simulink model "accBasedController_2015a"  (Simulink 8.5)
settings: Solver=ode45  SolverMode=SingleTasking  StartTime=0.0  StopTime=6  FixedStep=0.001  RelTol=1e-3
values from neighbouring files (symbols this model uses):
  A = [0 0 0 1 0 0;      0 0 0 0 1 0;      0 0 0 0 0 1;      -Ka/Jh Ka/Jh 0 0 0 0;     Ka/Je -(Ks + Ka)/Je Ks/Je 0 0 0;      0 Ks/Ja -Ks/Ja 0 0 -Beq/Ja]    [SimulationParam.m]    (also in SimulationParameters.m; abc_ws.mat = [0 0 0 1567.93947765 0 0 0 0 -1685.45584092 221.276595745 0 ; kalmanSS.m = [0 0 0 1 0 0;      0 0 0 0 1 0;      0 0 0 0 0 1;      -Ka/J; kalmanSSHumInput.m = [zeros(1,state_dim);      0 0 0 1 0;      0 0 0 0 1;      Ka)
  B = [zeros(3,control_dim); 1/Jh 0 0; 0 -1/Je 0; 0 0 N*KI/Ja]    [SimulationParam.m]    (also in SimulationParameters.m; abc_ws.mat = [1 0 0 0 0 0 0 0 -1.12996503145 0 0 0 ... (15 elements, 5x3); kalmanSS.m; kalmanSSHumInput.m = [1 0 0; zeros(2,control_dim); 0 -1/Je 0; 0 0 N*KI/Ja])
  Beq = 60    [SimulationParam.m]    (also in SimulationParameters.m; abc_ws.mat; kalmanSS.m; kalmanSSHumInput.m)
  C = [zeros(sensor_dim,state_dim)]    [SimulationParam.m]    (also in SimulationParameters.m; abc_ws.mat = [-1387.6 0 0 0 0 0 1387.6 0 1 0 0 0 ... (30 elements, 6x5)]; kalmanSS.m; kalmanSSHumInput.m)
  CURRENT_MAX = pi    (= 3.14159265359)    [SimulationParam.m]    (also in SimulationParameters.m; abc_ws.mat = 3.14)
  D = zeros(sensor_dim, control_dim)    [SimulationParam.m]    (also in SimulationParameters.m; abc_ws.mat = [0 1 0 0 0 0 0 0 0 0 0 0 ... (18 elements, 6x3)]; kalmanSS.m; kalmanSSHumInput.m = zeros(sensor_dim, control_dim); D(2,1) = 1)
  f = logspace(-2,2,1e4)    [kalmanSSHumInput.m]
  Ja = 0.47    [SimulationParam.m]    (also in SimulationParameters.m; abc_ws.mat; kalmanSS.m; kalmanSSHumInput.m)
  Je = W*Le^2    (= 0.88498313856)    [SimulationParam.m]    (also in SimulationParameters.m; abc_ws.mat; kalmanSS.m; kalmanSSHumInput.m)
  KI = 0.0603    [SimulationParam.m]    (also in SimulationParameters.m; abc_ws.mat; kalmanSS.m; kalmanSSHumInput.m)
  Le = 0.432    [SimulationParam.m]    (also in SimulationParameters.m; abc_ws.mat; kalmanSS.m; kalmanSSHumInput.m)
  N = 150    [SimulationParam.m]    (also in SimulationParameters.m; abc_ws.mat; kalmanSS.m; kalmanSSHumInput.m)
  Threaded_Ts = 0.001    [SimulationParam.m]    (also in SimulationParameters.m; abc_ws.mat)
  We = W*g    (= 46.5037717323)    [SimulationParam.m]    (also in SimulationParameters.m; abc_ws.mat; kalmanSS.m; kalmanSSHumInput.m)
libraries: simulink_extras x4, simulink x3, instrumentlib x2, eeGeneralControl x1
Description:
  | Collocated Admittance Control study for the acceleration-based SEA Transparency Control
settings Model: Creator=Leonardo Felipe  LastModifiedBy=leona  CovMetricSettings=dwe  CovHtmlReporting=off  covSaveCumulativeToWorkspaceVar=off  CovSaveSingleToWorkspaceVar=off  CovExternalEMLEnable=on
settings DataIOCC: MaxDataPoints=23000  SignalLoggingSaveFormat=Dataset  InspectSignalLogs=on
settings OptimizationCC: ExpressionDepthLimit=128
settings DebuggingCC: UnderspecifiedInitializationDetection=Simplified  MergeDetectMultiDrivingBlocksExec=error  FcnCallInpInsideContextMsg=EnableAllAsError  StateNameClashWarn=none  SFUnexpectedBacktrackingDiag=error  SFNoUnconditionalDefaultTransitionDiag=error
settings HardwareCC: ProdBitPerPointer=64  ProdLargestAtomicFloat=Float  ProdIntDivRoundTo=Zero  ProdEndianess=LittleEndian  ProdHWDeviceType=Specified
settings ModelReferenceCC: PropagateSignalLabelsOutOfModel=on
settings SFSimCC: SimUseLocalCustomCode=on
settings RTWCC: RTWUseLocalCustomCode=on
settings GRTTargetCC: TargetLangStandard=C99 (ISO)  CombineOutputUpdateFcns=on  GRTInterface=off

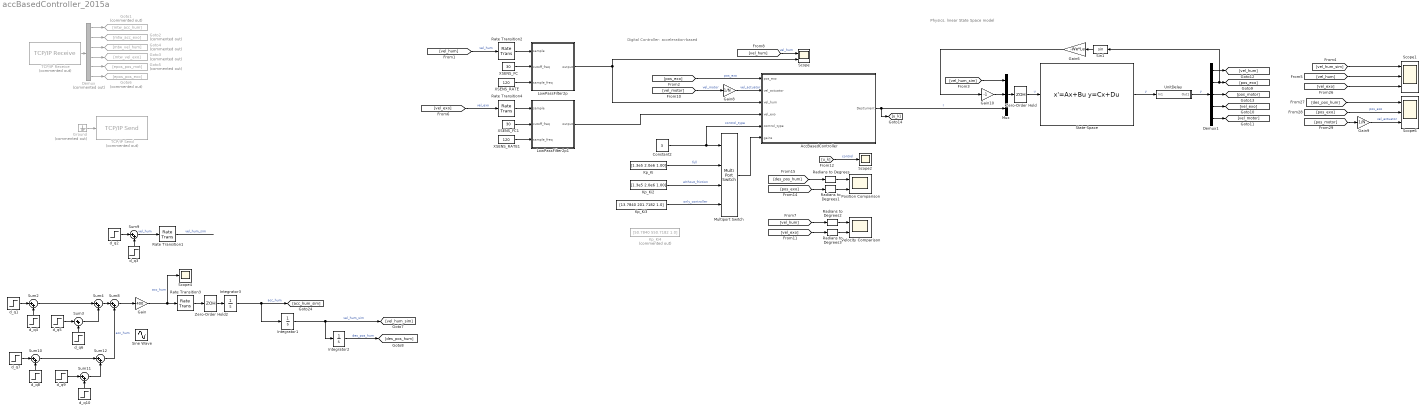
== system accBasedController_2015a ==
  note: Digital Controller: acceleration-based
  note: Physics, linear State Space model
  AccBasedController : Subsystem
  Constant2 : Constant  Value=3
  Demux : Demux  Commented=on  Outputs=6
  Demux1 : Demux  Outputs=5
  Gain : Gain  Gain=400
  Gain10 : Gain  Gain=-1
  Gain6 : Gain  Gain=-We*Le
  Gain8 : Gain  Gain=1/N
  Gain9 : Gain  Gain=1/N
  Goto1 : Goto  Commented=on  GotoTag=mtw_acc_hum
  Goto2 : Goto  Commented=on  GotoTag=mtw_acc_exo
  Goto3 : Goto  Commented=on  GotoTag=mtw_vel_exo
  Goto4 : Goto  Commented=on  GotoTag=mtw_vel_hum
  Goto5 : Goto  Commented=on  GotoTag=epos_pos_mot
  Goto6 : Goto  Commented=on  GotoTag=epos_pos_exo
  Ground : Ground  Commented=on
  Integrator1 : Integrator
  Integrator2 : Integrator
  Integrator3 : Integrator
  Kp_Ki : Constant  Value=[1.3e5 2.0e6 1.00]
  Kp_Ki2 : Constant  Value=[1.3e5 2.0e6 1.00]
  Kp_Ki3 : Constant  Value=[13.7840 201.7182 1.0]
  Kp_Ki4 : Constant  Commented=on  Value=[50.7840 550.7182 1.0]
  LowPassFilter2p : Subsystem
  LowPassFilter2p1 : Subsystem
  Multiport Switch : MultiPortSwitch
  Mux : Mux  Inputs=3
  Position Comparison : Scope  NumInputPorts=2
      settings: TimeRange=auto  MaxDataPoints=5000  SaveToWorkspace=off  YMin=-3.29771~-5  YMax=29.67935~5  SampleTime=-1
  Radians to Degrees{,1..3} (4 alike) : simulink_extras/Transformations/Radians to Degrees
  Rate Transition1 : RateTransition  OutPortSampleTime=Threaded_Ts
  Rate Transition2 : RateTransition  OutPortSampleTime=0.008
  Rate Transition3 : RateTransition  OutPortSampleTime=Threaded_Ts
  Rate Transition4 : RateTransition  OutPortSampleTime=0.008
  Scope : Scope  NumInputPorts=2
      settings: TimeRange=auto  MaxDataPoints=5000  SaveToWorkspace=off  SaveName=ScopeData2  YMin=-0.03282~-5  YMax=0.26283~5  SampleTime=-1
  Scope1 : Scope  NumInputPorts=3
      settings: TimeRange=auto  MaxDataPoints=5000  SaveToWorkspace=off  YMin=-0.01455~-5~-5  YMax=0.24273~5~5  SampleTime=-1
  Scope2 : Scope
      settings: TimeRange=auto  MaxDataPoints=5000  SaveToWorkspace=off  YMin=-3.925  YMax=3.925  SampleTime=-1
  Scope4 : Scope
      settings: TimeRange=auto  MaxDataPoints=5000  SaveToWorkspace=off  SaveName=ScopeData4  YMin=-50.00000  YMax=50.00000  SampleTime=-1
  Scope6 : Scope  NumInputPorts=3
      settings: TimeRange=auto  ShowLegends=on  MaxDataPoints=5000  SaveToWorkspace=off  YMin=-0.05756~-5~-5  YMax=0.518~5~5  SampleTime=-1
  Sin1 : Trigonometry
  Sine Wave : Sin  SampleTime=0
  State-Space : StateSpace  A=A  B=B  C=C  D=D  X0=0  ContinuousStateAttributes={'x_h','x_e','x_a','dx_e','dx_a'}
  Sum{2..4,8..12} (8 alike) : Sum  Inputs=|++
  TCP/IP Receive : instrumentlib/TCP//IP Receive  Commented=on  Host=127.0.0.1  Port=23000  DataSize="[1  6]"  EnableBlockingMode=on  Timeout=0.3  SampleTime=Threaded_Ts  DataType=single  ByteOrder=BigEndian  ASCIIFormatting=%f,  Terminator=LF
  TCP/IP Send : instrumentlib/TCP//IP Send  Commented=on  Host=127.0.0.1  Port=23001  EnableBlockingMode=on  Timeout=0.3  ByteOrder=BigEndian  TransferDelay=off
  UnitDelay : Subsystem  TreatAsAtomicUnit=on  SystemSampleTime=Threaded_Ts
  Velocity Comparison : Scope  NumInputPorts=2
      settings: TimeRange=auto  MaxDataPoints=5000  SaveToWorkspace=off  SaveName=ScopeData2  YMin=-7.82186~-5  YMax=13.60083~5  SampleTime=-1
  XSENS_FC : Constant  Value=30
  XSENS_FC1 : Constant  Value=30
  XSENS_RATE : Constant  Value=120
  XSENS_RATE1 : Constant  Value=120
  Zero-Order Hold : ZeroOrderHold  SampleTime=Threaded_Ts
  Zero-Order Hold2 : ZeroOrderHold  SampleTime=Threaded_Ts
  d_q1 : Step  Time=0.76  SampleTime=0.008
  d_q10 : Step  Time=2.808  After=-1  SampleTime=0.008
  d_q2 : Step  SampleTime=0.008
  d_q3 : Step  Time=1.4  After=-1  SampleTime=0.008
  d_q4 : Step  Time=0.784  After=-1  SampleTime=0.008
  d_q5 : Step  Time=0.784  After=-1  SampleTime=0.008
  d_q6 : Step  Time=0.808  SampleTime=0.008
  d_q7 : Step  Time=2.76  After=-1  SampleTime=0.008
  d_q8 : Step  Time=2.784  SampleTime=0.008
  d_q9 : Step  Time=2.784  SampleTime=0.008
  wires:
  d_q3/1 -> Sum9/2
  d_q2/1 -> Sum9/1
  Sum9/1 -> Rate Transition1/1  "vel_hum"
  TCP/IP Receive/1 -> Demux/1
  Demux/1 -> Goto1/1
  Demux/2 -> Goto2/1
  Demux/3 -> Goto4/1
  Demux/4 -> Goto3/1
  Demux/5 -> Goto5/1
  Demux/6 -> Goto6/1
  Ground/1 -> TCP/IP Send/1
  Integrator1/1 -> Integrator2/1, [vel_hum_sim]  "vel_hum_sim"
  Integrator2/1 -> [des_pos_hum]  "des_pos_hum"
  Zero-Order Hold/1 -> State-Space/1  "u"
  State-Space/1 -> UnitDelay/1(In1)  "y"
  [vel_hum_sim] -> Mux/1
  Mux/1 -> Zero-Order Hold/1
  Demux1/5 -> [vel_motor]
  Demux1/1 -> [vel_hum]
  UnitDelay/1(Out1) -> Demux1/1  "y"
  [vel_hum_sim] -> Scope1/1
  [vel_hum] -> Scope1/2
  [vel_hum] -> Radians to Degrees2/1
  [vel_exo] -> Radians to Degrees3/1
  [des_pos_hum] -> Radians to Degrees/1
  [pos_exo] -> Radians to Degrees1/1
  d_q1/1 -> Sum2/1
  d_q4/1 -> Sum2/2
  d_q6/1 -> Sum3/2
  d_q5/1 -> Sum3/1
  Sum2/1 -> Sum4/1
  Sum3/1 -> Sum4/2
  Sum8/1 -> Gain/1
  Rate Transition1/1 -> ?  "vel_hum_sim"
  Zero-Order Hold2/1 -> Integrator3/1
  Integrator3/1 -> Integrator1/1, [acc_hum_sim]  "acc_hum"
  Rate Transition3/1 -> Zero-Order Hold2/1
  Sum11/1 -> Sum12/2
  Sum10/1 -> Sum12/1
  d_q9/1 -> Sum11/1
  d_q10/1 -> Sum11/2
  d_q8/1 -> Sum10/2
  d_q7/1 -> Sum10/1
  Sum4/1 -> Sum8/1
  Sum12/1 -> Sum8/2  "acc_hum"
  [vel_exo] -> Scope1/3
  [des_pos_hum] -> Scope6/1
  [pos_exo] -> Scope6/2  "pos_exo"
  Gain/1 -> Rate Transition3/1, Scope4/1  "acc_hum"
  Kp_Ki/1 -> Multiport Switch/2  "full"
  Kp_Ki2/1 -> Multiport Switch/3  "without_friction"
  Kp_Ki3/1 -> Multiport Switch/4  "only_controller"
  Constant2/1 -> AccBasedController/5(control_type), Multiport Switch/1  "control_type"
  [pos_exo] -> AccBasedController/1(pos_exo)  "pos_exo"
  [vel_motor] -> Gain8/1  "vel_motor"
  Multiport Switch/1 -> AccBasedController/6(gains)
  Sin1/1 -> Gain6/1
  Demux1/2 -> Sin1/1, [pos_exo]
  AccBasedController/1(DesCurrent) -> Mux/3, [u_k]  "I"
  Gain6/1 -> Gain10/1
  Demux1/3 -> [pos_motor]
  Demux1/4 -> [vel_exo]
  Gain8/1 -> AccBasedController/2(vel_actuator)  "vel_actuator"
  [pos_motor] -> Gain9/1
  Gain9/1 -> Scope6/3  "vel_actuator"
  Radians to Degrees/1 -> Position Comparison/1
  Radians to Degrees1/1 -> Position Comparison/2
  Radians to Degrees2/1 -> Velocity Comparison/1
  Radians to Degrees3/1 -> Velocity Comparison/2
  [u_k] -> Scope2/1  "control"
  Gain10/1 -> Mux/2
  Rate Transition2/1 -> LowPassFilter2p/1(sample)
  XSENS_RATE/1 -> LowPassFilter2p/3(sample_freq)
  XSENS_FC/1 -> LowPassFilter2p/2(cutoff_freq)
  [vel_hum] -> Scope/1  "vel_hum"
  [vel_hum] -> Rate Transition2/1  "vel_hum"
  LowPassFilter2p/1(output) -> AccBasedController/3(vel_hum), Scope/2
  XSENS_FC1/1 -> LowPassFilter2p1/2(cutoff_freq)
  XSENS_RATE1/1 -> LowPassFilter2p1/3(sample_freq)
  Rate Transition4/1 -> LowPassFilter2p1/1(sample)
  [vel_exo] -> Rate Transition4/1  "vel_exo"
  LowPassFilter2p1/1(output) -> AccBasedController/4(vel_exo)

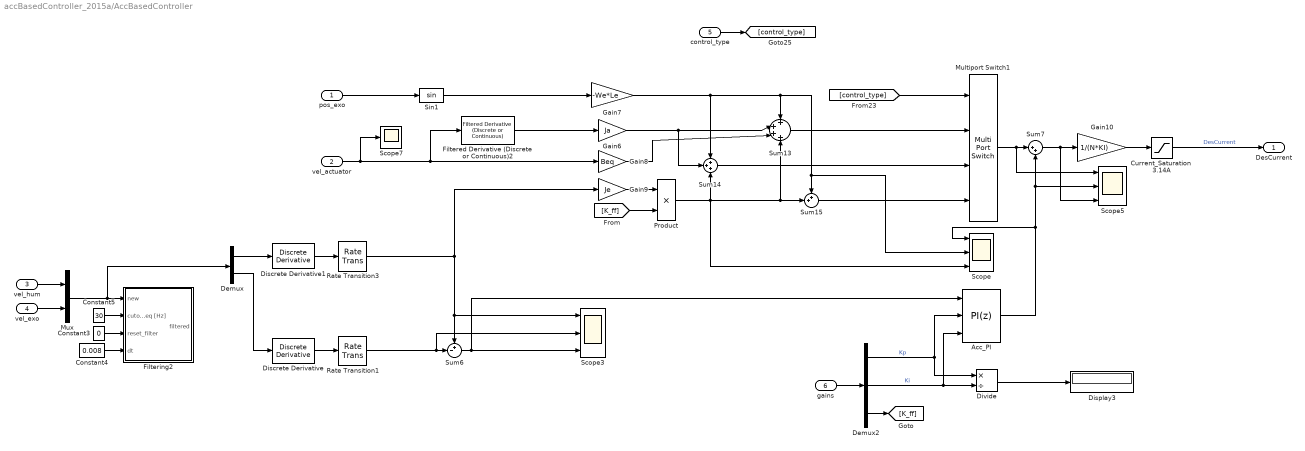
== system accBasedController_2015a/AccBasedController ==
  pos_exo : Inport
  vel_actuator : Inport  Port=2
  vel_hum : Inport  Port=3
  vel_exo : Inport  Port=4
  control_type : Inport  Port=5
  gains : Inport  Port=6
  Acc_PI : simulink/Continuous/PID Controller  Controller=PI  Form=Parallel  TimeDomain=Discrete-time  SampleTime=Threaded_Ts  IntegratorMethod=Forward Euler  FilterMethod=Forward Euler  ControllerParametersSource=external  P=13.7840  I=101.7182  D=0  UseFilter=on  N=100  InitialConditionSource=internal  InitialConditionForIntegrator=0  InitialConditionForFilter=0  DifferentiatorICPrevScaledInput=0  ExternalReset=none  TrackingMode=off  Kt=1  LimitOutput=off  UpperSaturationLimit=inf  LowerSaturationLimit=-inf  LinearizeAsGain=on  AntiWindupMode=none  Kb=1  POutMin=[]  POutMax=[]  IOutMin=[]  IOutMax=[]  DOutMin=[]  DOutMax=[]  NOutMin=[]  NOutMax=[]  SumOutMin=[]  SumOutMax=[]  SaturationOutMin=[]  SaturationOutMax=[]  PParamMin=[]  PParamMax=[]  IParamMin=[]  IParamMax=[]  DParamMin=[]  DParamMax=[]  NParamMin=[]  NParamMax=[]  KbParamMin=[]  KbParamMax=[]  KtParamMin=[]  KtParamMax=[]  KbOutMin=[]  KbOutMax=[]  KtOutMin=[]  KtOutMax=[]  IntegratorOutMin=[]  IntegratorOutMax=[]  FilterOutMin=[]  FilterOutMax=[]  SumI1OutMin=[]  SumI1OutMax=[]  SumI2OutMin=[]  SumI2OutMax=[]  SumI3OutMin=[]  SumI3OutMax=[]  SumDOutMin=[]  SumDOutMax=[]  DifferentiatorOutMin=[]  DifferentiatorOutMax=[]  IntegratorContinuousStateAttributes=''  IntegratorStateMustResolveToSignalObject=off  IntegratorRTWStateStorageClass=Auto  FilterContinuousStateAttributes=''  FilterStateMustResolveToSignalObject=off  FilterRTWStateStorageClass=Auto
  Constant3 : Constant  Value=0
  Constant4 : Constant  Value=0.008
  Constant5 : Constant  Value=30
  Current_Saturation  3.14A : Saturate  UpperLimit=CURRENT_MAX  LowerLimit=-CURRENT_MAX
  Demux : Demux  Outputs=2
  Demux2 : Demux  Outputs=3
  Discrete Derivative : simulink/Discrete/Discrete Derivative  gainval=1.0  ICPrevScaledInput=0.0  OutMin=[]  OutMax=[]  OutDataType=fixdt(1, 16)  OutScaling=2^-10  DoSatur=off
  Discrete Derivative1 : simulink/Discrete/Discrete Derivative  gainval=1.0  ICPrevScaledInput=0.0  OutMin=[]  OutMax=[]  OutDataType=fixdt(1, 16)  OutScaling=2^-10  DoSatur=off
  Display3 : Display
  Divide : Product  Inputs=*/
  Filtered Derivative (Discrete or Continuous)2 : eeGeneralControl/Filtered Derivative (Discrete or Continuous)  K=1  T=0.01  B=10000  A=-10000  minRatio=10  init_option=Inherited from block input  x0=0  Ts=Threaded_Ts
  Filtering2 : Subsystem
  Gain10 : Gain  Gain=1/(N*KI)
  Gain6 : Gain  Gain=Ja
  Gain7 : Gain  Gain=-We*Le
  Gain8 : Gain  Gain=Beq
  Gain9 : Gain  Gain=Je
  Multiport Switch1 : MultiPortSwitch
  Mux : Mux  Inputs=2
  Product : Product
  Rate Transition1 : RateTransition  OutPortSampleTime=0.001
  Rate Transition3 : RateTransition  OutPortSampleTime=0.001
  Scope : Scope  NumInputPorts=3
      settings: TimeRange=auto  MaxDataPoints=5000  SaveToWorkspace=off  YMin=-163.16281~-5~-5  YMax=184.21692~5~5  SampleTime=-1
  Scope3 : Scope  NumInputPorts=3
      settings: TimeRange=auto  MaxDataPoints=5000  SaveToWorkspace=off  SaveName=ScopeData3  YMin=-9.48144~-5~-5  YMax=9.47721~5~5  SampleTime=-1
  Scope5 : Scope  NumInputPorts=3
      settings: TimeRange=auto  MaxDataPoints=5000  SaveToWorkspace=off  YMin=-21.74461~-5~-5  YMax=29.12285~5~5  SampleTime=-1
  Scope7 : Scope
      settings: TimeRange=auto  MaxDataPoints=5000  SaveToWorkspace=off  SaveName=ScopeData2  YMin=-0.64032  YMax=0.59663  SampleTime=-1
  Sin1 : Trigonometry
  Sum13 : Sum  Inputs=++++
  Sum14 : Sum  Inputs=+++
  Sum15 : Sum  Inputs=++|
  Sum6 : Sum  Inputs=+-|
  Sum7 : Sum  Inputs=|++
  DesCurrent : Outport
  wires:
  Gain7/1 -> Scope/2, Sum15/1, Sum13/1, Sum14/1
  Gain6/1 -> Sum13/2, Sum14/2
  Product/1 -> Scope/3, Sum15/2, Sum13/4, Sum14/3
  Gain10/1 -> Current_Saturation  3.14A/1
  Sum7/1 -> Scope5/3, Gain10/1
  Demux2/1 -> Divide/1, Acc_PI/2  "Kp"
  Gain8/1 -> Sum13/3
  Rate Transition3/1 -> Gain9/1, Sum6/1, Scope3/1
  Demux2/2 -> Acc_PI/3, Divide/2  "Ki"
  pos_exo/1 -> Sin1/1
  Multiport Switch1/1 -> Scope5/1, Sum7/1
  Divide/1 -> Display3/1
  vel_actuator/1 -> Scope7/1, Filtered Derivative (Discrete or Continuous)2/1, Gain8/1
  [control_type] -> Multiport Switch1/1
  Sum13/1 -> Multiport Switch1/2
  Sin1/1 -> Gain7/1
  control_type/1 -> [control_type]
  Sum14/1 -> Multiport Switch1/3
  Sum15/1 -> Multiport Switch1/4
  Filtered Derivative (Discrete or Continuous)2/1 -> Gain6/1
  Discrete Derivative/1 -> Rate Transition1/1
  Current_Saturation  3.14A/1 -> DesCurrent/1  "DesCurrent"
  gains/1 -> Demux2/1
  Sum6/1 -> Acc_PI/1, Scope3/3
  Demux2/3 -> [K_ff]
  [K_ff] -> Product/2
  Gain9/1 -> Product/1
  Acc_PI/1 -> Scope/1, Sum7/2, Scope5/2
  Rate Transition1/1 -> Sum6/2, Scope3/2
  Constant4/1 -> Filtering2/4(dt)
  Constant5/1 -> Filtering2/2(cutoff_freq [Hz])
  Constant3/1 -> Filtering2/3(reset_filter)
  Discrete Derivative1/1 -> Rate Transition3/1
  vel_hum/1 -> Mux/1
  vel_exo/1 -> Mux/2
  Mux/1 -> Demux/1, Filtering2/1(new)
  Demux/1 -> Discrete Derivative1/1
  Demux/2 -> Discrete Derivative/1

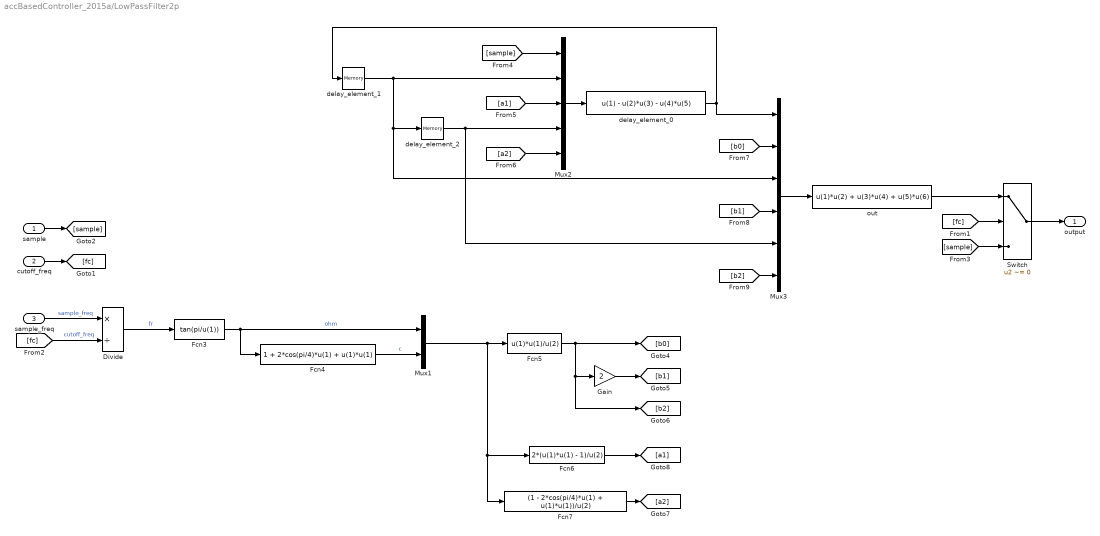
== system accBasedController_2015a/LowPassFilter2p ==
  sample : Inport
  cutoff_freq : Inport  Port=2
  sample_freq : Inport  Port=3
  Divide : Product  Inputs=*/
  Fcn3 : Fcn  Expr=tan(pi/u(1))
  Fcn4 : Fcn  Expr=1 + 2*cos(pi/4)*u(1) + u(1)*u(1)
  Fcn5 : Fcn  Expr=u(1)*u(1)/u(2)
  Fcn6 : Fcn  Expr=2*(u(1)*u(1) - 1)/u(2)
  Fcn7 : Fcn  Expr=(1 - 2*cos(pi/4)*u(1) + u(1)*u(1))/u(2)
  Gain : Gain  Gain=2
  Mux1 : Mux  Inputs=2
  Mux2 : Mux  Inputs=5
  Mux3 : Mux  Inputs=6
  Switch : Switch  Criteria=u2 ~= 0
  delay_element_0 : Fcn  Expr=u(1) - u(2)*u(3) - u(4)*u(5)
  delay_element_1 : Memory  InheritSampleTime=on
  delay_element_2 : Memory  InheritSampleTime=on
  out : Fcn  Expr=u(1)*u(2) + u(3)*u(4) + u(5)*u(6)
  output : Outport
  wires:
  Switch/1 -> output/1
  cutoff_freq/1 -> [fc]
  [fc] -> Switch/2
  sample_freq/1 -> Divide/1  "sample_freq"
  [fc] -> Divide/2  "cutoff_freq"
  Divide/1 -> Fcn3/1  "fr"
  Mux1/1 -> Fcn7/1, Fcn6/1, Fcn5/1
  Fcn3/1 -> Mux1/1, Fcn4/1  "ohm"
  Fcn4/1 -> Mux1/2  "c"
  Fcn5/1 -> [b0], [b2], Gain/1
  Gain/1 -> [b1]
  Fcn6/1 -> [a1]
  Fcn7/1 -> [a2]
  sample/1 -> [sample]
  [sample] -> Switch/3
  delay_element_1/1 -> delay_element_2/1, Mux3/3, Mux2/2
  [sample] -> Mux2/1
  Mux2/1 -> delay_element_0/1
  [a1] -> Mux2/3
  delay_element_2/1 -> Mux2/4, Mux3/5
  [a2] -> Mux2/5
  out/1 -> Switch/1
  delay_element_0/1 -> delay_element_1/1, Mux3/1
  [b0] -> Mux3/2
  [b1] -> Mux3/4
  [b2] -> Mux3/6
  Mux3/1 -> out/1

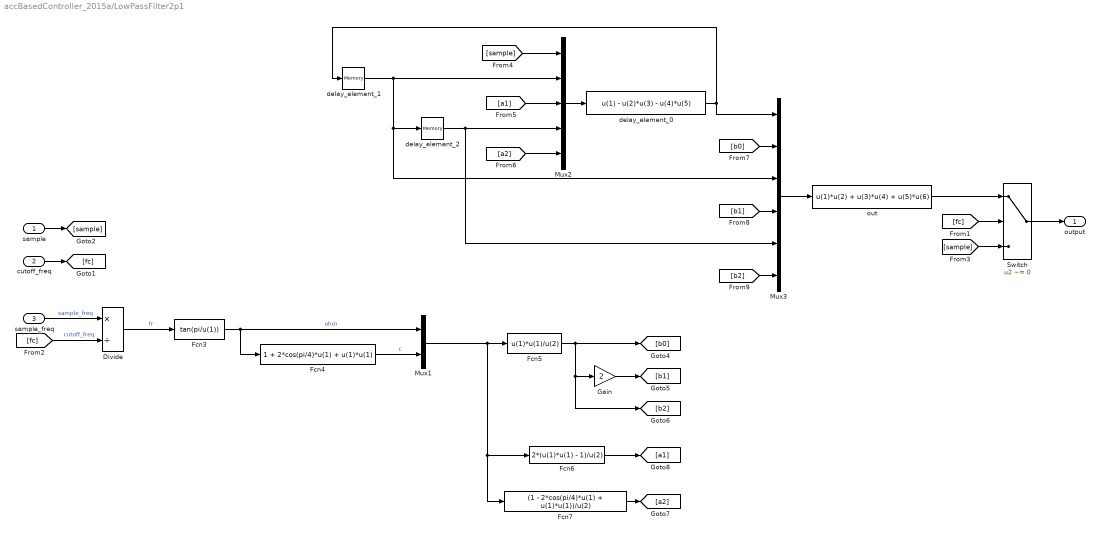
== system accBasedController_2015a/LowPassFilter2p1 ==
  sample : Inport
  cutoff_freq : Inport  Port=2
  sample_freq : Inport  Port=3
  Divide : Product  Inputs=*/
  Fcn3 : Fcn  Expr=tan(pi/u(1))
  Fcn4 : Fcn  Expr=1 + 2*cos(pi/4)*u(1) + u(1)*u(1)
  Fcn5 : Fcn  Expr=u(1)*u(1)/u(2)
  Fcn6 : Fcn  Expr=2*(u(1)*u(1) - 1)/u(2)
  Fcn7 : Fcn  Expr=(1 - 2*cos(pi/4)*u(1) + u(1)*u(1))/u(2)
  Gain : Gain  Gain=2
  Mux1 : Mux  Inputs=2
  Mux2 : Mux  Inputs=5
  Mux3 : Mux  Inputs=6
  Switch : Switch  Criteria=u2 ~= 0
  delay_element_0 : Fcn  Expr=u(1) - u(2)*u(3) - u(4)*u(5)
  delay_element_1 : Memory  InheritSampleTime=on
  delay_element_2 : Memory  InheritSampleTime=on
  out : Fcn  Expr=u(1)*u(2) + u(3)*u(4) + u(5)*u(6)
  output : Outport
  wires:
  Mux3/1 -> out/1
  [b2] -> Mux3/6
  [b1] -> Mux3/4
  [b0] -> Mux3/2
  delay_element_0/1 -> Mux3/1, delay_element_1/1
  out/1 -> Switch/1
  [a2] -> Mux2/5
  delay_element_2/1 -> Mux3/5, Mux2/4
  [a1] -> Mux2/3
  Mux2/1 -> delay_element_0/1
  [sample] -> Mux2/1
  delay_element_1/1 -> Mux2/2, Mux3/3, delay_element_2/1
  [sample] -> Switch/3
  sample/1 -> [sample]
  Fcn7/1 -> [a2]
  Fcn6/1 -> [a1]
  Gain/1 -> [b1]
  Fcn5/1 -> Gain/1, [b2], [b0]
  Fcn4/1 -> Mux1/2  "c"
  Fcn3/1 -> Fcn4/1, Mux1/1  "ohm"
  Mux1/1 -> Fcn5/1, Fcn6/1, Fcn7/1
  Divide/1 -> Fcn3/1  "fr"
  [fc] -> Divide/2  "cutoff_freq"
  sample_freq/1 -> Divide/1  "sample_freq"
  [fc] -> Switch/2
  cutoff_freq/1 -> [fc]
  Switch/1 -> output/1

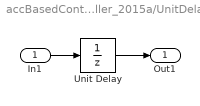
== system accBasedController_2015a/UnitDelay ==
  In1 : Inport
  Unit Delay : UnitDelay  SampleTime=-1  HasFrameUpgradeWarning=on
  Out1 : Outport
  wires:
  Unit Delay/1 -> Out1/1
  In1/1 -> Unit Delay/1

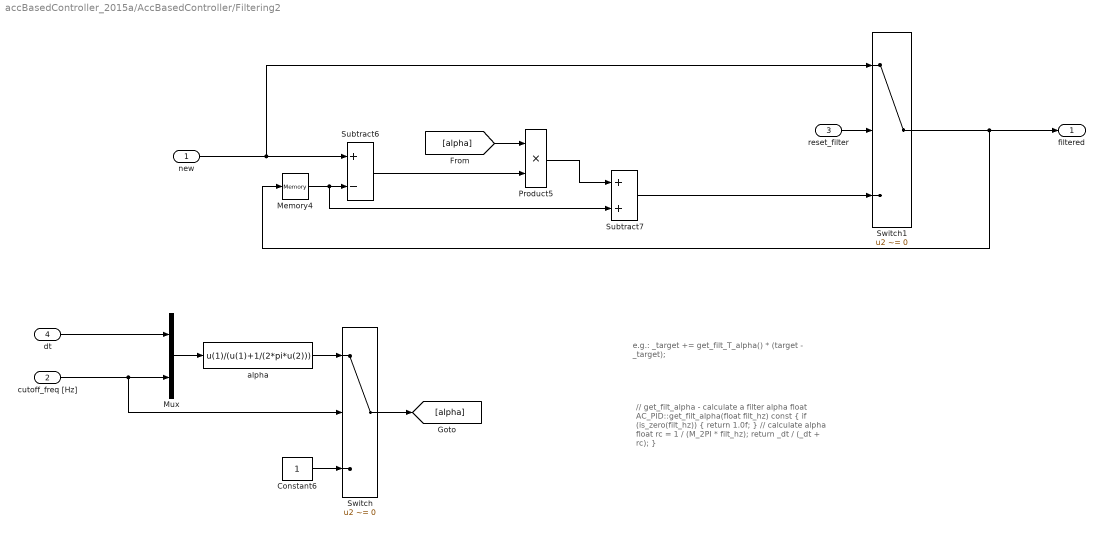
== system accBasedController_2015a/AccBasedController/Filtering2 ==
  note: e.g.:
      |
      | _target += get_filt_T_alpha() * (target - _target);
  note: // get_filt_alpha - calculate a filter alpha
      | float AC_PID::get_filt_alpha(float filt_hz) const
      | {
      |     if (is_zero(filt_hz)) {
      |         return 1.0f;
      |     }
      |
      |     // calculate alpha
      |     float rc = 1 / (M_2PI * filt_hz);
      |     return _dt / (_dt + rc);
      | }
  new : Inport
  cutoff_freq [Hz] : Inport  Port=2
  reset_filter : Inport  Port=3
  dt : Inport  Port=4
  Constant6 : Constant
  Memory4 : Memory  InheritSampleTime=on
  Mux : Mux  Inputs=2
  Product5 : Product
  Subtract6 : Sum  Inputs=+-
  Subtract7 : Sum
  Switch : Switch  Criteria=u2 ~= 0
  Switch1 : Switch  Criteria=u2 ~= 0
  alpha : Fcn  Expr=u(1)/(u(1)+1/(2*pi*u(2)))
  filtered : Outport
  wires:
  dt/1 -> Mux/1
  alpha/1 -> Switch/1
  cutoff_freq [Hz]/1 -> Mux/2, Switch/2
  Mux/1 -> alpha/1
  Product5/1 -> Subtract7/1
  Subtract6/1 -> Product5/2
  Memory4/1 -> Subtract7/2, Subtract6/2
  new/1 -> Switch1/1, Subtract6/1
  Constant6/1 -> Switch/3
  Switch/1 -> [alpha]
  [alpha] -> Product5/1
  reset_filter/1 -> Switch1/2
  Switch1/1 -> filtered/1, Memory4/1
  Subtract7/1 -> Switch1/3
